simulink model "project_Auto_final"  (R2023b)
settings: Solver=FixedStepAuto  StartTime=0.0  StopTime=inf  FixedStep=0.01  RelTol=1e-3
values from neighbouring files (symbols this model uses):
  den_Gd = Gd.Den{:}    [para.m]
  encoder_scale = 1/12/4 *2*pi    (= 0.1308996939)    [para.m]
  KD = 0    [para.m]
  KI = 0.25    [para.m]
  KP = 0.05    [para.m]
  num_Gd = Gd.Num{:}    [para.m]
  Ts = 1e-2    (= 0.01)    [para.m]
  Vlim = 12    [para.m]
  Wref = 300    [para.m]
libraries: arduinolib x10, arduinosensorlib x5, simulink x2
settings Model: SimulationMode=external  ExtModeTrigDuration=2  Creator=wj671  LastModifiedBy=wj671
settings OptimizationCC: EnhancedBackFolding=on  PassReuseOutputArgsAs=Individual arguments  ZeroExternalMemoryAtStartup=off  ZeroInternalMemoryAtStartup=off  MaxStackSize=64  OptimizeBlockOrder=speed  DifferentSizesBufferReuse=on  OptimizationCustomize=off  EfficientTunableParamExpr=on
settings DebuggingCC: ParameterTunabilityLossMsg=error
settings HardwareCC: ProdBitPerInt=16  ProdBitPerPointer=16  ProdBitPerSizeT=16  ProdBitPerPtrDiffT=16  ProdLargestAtomicFloat=None  ProdWordSize=8  ProdHWDeviceType=Atmel->AVR
settings SFSimCC: MATLABDynamicMemAlloc=off
settings RTWCC: Description=Embedded Coder  SystemTargetFile=ert.tlc  HardwareBoard=Arduino Mega 2560  TemplateMakefile=ert_default_tmf  Toolchain=Arduino AVR  BuildConfiguration=Faster Runs
settings CodeAppCC: ForceParamTrailComments=on  IgnoreCustomStorageClasses=off  OperatorAnnotations=on  SimulinkDataObjDesc=on  SFDataObjDesc=on  InsertBlockDesc=on
settings ERTTargetCC: SupportContinuousTime=on  SupportVariableSizeSignals=on  ExtMode=on  ExtModeTransport=3  ExtModeStaticAlloc=on  ExtModeAutomaticAllocSize=off  ExtModeStaticAllocSize=2048  ExtModeMexFile=ext_xcp  ExtModeMexArgs=0 8 921600  ExtModeIntrfLevel=Level2 - Open

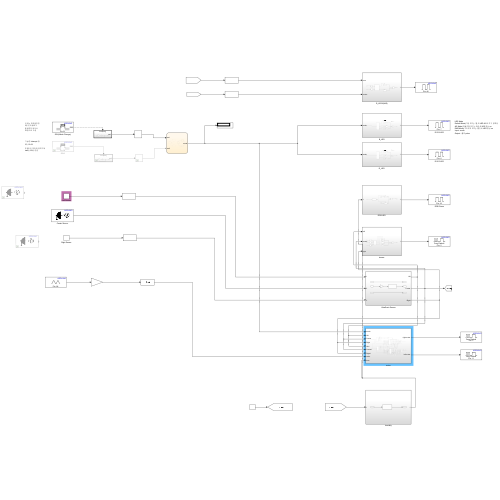
[thumbnail: Simulink's stored preview of the top-level diagram]
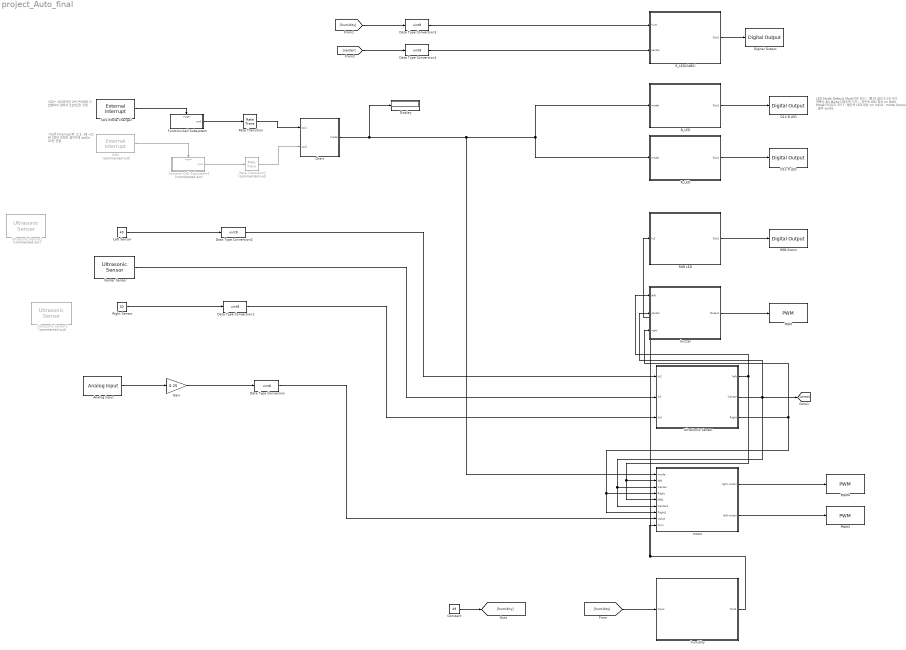
== system project_Auto_final ==
  note: 이유는 모르겠지만 2번 인터럽트가
      | 발생하지 않아서
      | 21번으로 수정
  note: 가능한 Interrupt 핀:
      | 2,3, 18~21
      |
      | 핀 3번이 모터와 겹치기에
      | sw2는 20번 연결
  note: LED Mode
      | Default Mode(기본 모드) : 빨,파 LED 0.2초 주기 깜빡임
      | AD Mode(자율주행 모드) : 파란색 LED 항상 on
      | DMS Mode(거리유지 모드) : 빨간색 LED 항상 on
      | Input : mode
      | Output : 출력 pulse
  Analog Input : arduinolib/Analog Input  pinNumber=2  ReadResultsOnly=off  ConversionTriggerSource=Software  ExternalTriggerType=uint32( 0 )  OutputDataType=uint16  EnableConversionCompleteNotify=off  EnableOuputStatus=off  SampleTime=-1  blockPlatform=arduino
  B_LED : Subsystem
  Center Sensor : arduinosensorlib/Ultrasonic Sensor  NumSignalPins=2  TrigPin=32  EchoPin=33  SignalPin=3  SampleTime_=0.1  blockPlatform=ARDUINO
  Chart : Stateflow chart  TreatAsAtomicUnit=on
  Constant : Constant  Value=49
  D12 R LED : arduinolib/Digital Output  pinNumber=6  Direction=output  blockPlatform=arduino
  D13 B LED : arduinolib/Digital Output  pinNumber=7  Direction=output  blockPlatform=arduino
  Data Type Conversion{,1..4} (5 alike) : DataTypeConversion  OutDataTypeStr=uint8  SaturateOnIntegerOverflow=off  RndMeth=Floor
  Digital Output : arduinolib/Digital Output  pinNumber=46  Direction=output  blockPlatform=arduino
  Display : Display
  Function-Call Subsystem : Subsystem  TreatAsAtomicUnit=on
  Function-Call Subsystem1 : Subsystem  Commented=on  TreatAsAtomicUnit=on
  Gain : Gain  Gain=0.25
  Left Sensor : Constant  Value=40
  PWM : arduinolib/PWM  pinNumber=5  frequencyType=Default  desiredFrequency=490.2  achievableFrequency=490.2
  PWM3 : arduinolib/PWM  pinNumber=11  frequencyType=Default  desiredFrequency=490.2  achievableFrequency=490.2
  PWM4 : arduinolib/PWM  pinNumber=3  frequencyType=Default  desiredFrequency=490.2  achievableFrequency=490.2
  RGB Grenn : arduinolib/Digital Output  pinNumber=10  Direction=output  blockPlatform=arduino
  RGB LED : Subsystem
  R_LED : Subsystem
  R_LED2(ABS) : Subsystem
  Rate Transition : RateTransition  Integrity=off  OutPortSampleTime=0.05
  Rate Transition1 : RateTransition  Commented=on  Integrity=off  OutPortSampleTime=0.05
  Right Sensor : Constant  Value=40
  SW1(Mode Change) : arduinolib/External Interrupt  Pin=21  PullUp=off  Mode=FALLING  InterruptSimulationInput=off
  SW2 : arduinolib/External Interrupt  Commented=on  Pin=20  PullUp=off  Mode=FALLING  InterruptSimulationInput=off
  UltraSonic Sensor : Subsystem
  Ultrasonic Sensor1 : arduinosensorlib/Ultrasonic Sensor  Commented=on  NumSignalPins=2  TrigPin=42  EchoPin=43  SignalPin=3  SampleTime_=0.1  blockPlatform=ARDUINO
  Ultrasonic Sensor2 : arduinosensorlib/Ultrasonic Sensor  Commented=on  NumSignalPins=2  TrigPin=50  EchoPin=51  SignalPin=3  SampleTime_=0.1  blockPlatform=ARDUINO
  buzzer : Subsystem
  humidity : Subsystem
  motor : Subsystem
  wires:
  R_LED/1(Out1) -> D12 R LED/1
  Rate Transition/1 -> Chart/1(sw1)
  B_LED/1(Out1) -> D13 B LED/1
  SW1(Mode Change)/1 -> Function-Call Subsystem/Trigger
  Function-Call Subsystem/1(sw1) -> Rate Transition/1
  Chart/1(mode) -> Display/1, motor/1(mode), B_LED/1(mode), R_LED/1(mode)
  Center Sensor/1 -> UltraSonic Sensor/2(In1)
  Left Sensor/1 -> Data Type Conversion2/1
  Right Sensor/1 -> Data Type Conversion1/1
  UltraSonic Sensor/3(Right) -> buzzer/3(right), motor/7(Right1), motor/4(Right)
  UltraSonic Sensor/1(left) -> buzzer/1(left), motor/5(left1), motor/2(left)
  UltraSonic Sensor/2(Center) -> [center], buzzer/2(center), motor/6(Center1), motor/3(Center)
  motor/1(right motor) -> PWM4/1
  motor/2(left motor) -> PWM3/1
  Data Type Conversion1/1 -> UltraSonic Sensor/3(In3)
  Data Type Conversion2/1 -> UltraSonic Sensor/1(In2)
  Function-Call Subsystem1/1(sw2) -> Rate Transition1/1
  Rate Transition1/1 -> Chart/2(sw2)
  SW2/1 -> Function-Call Subsystem1/Trigger
  Gain/1 -> Data Type Conversion/1
  Analog Input/1 -> Gain/1
  Data Type Conversion/1 -> motor/8(value)
  humidity/1(Out1) -> RGB LED/1(In2), motor/9(hum)
  RGB LED/1(Out1) -> RGB Grenn/1
  buzzer/1(Output) -> PWM/1
  Constant/1 -> [humidity]
  [humidity] -> humidity/1(Input)
  [humidity] -> Data Type Conversion3/1
  [center] -> Data Type Conversion4/1
  R_LED2(ABS)/1(Out1) -> Digital Output/1
  Data Type Conversion3/1 -> R_LED2(ABS)/1(hum)
  Data Type Conversion4/1 -> R_LED2(ABS)/2(center)

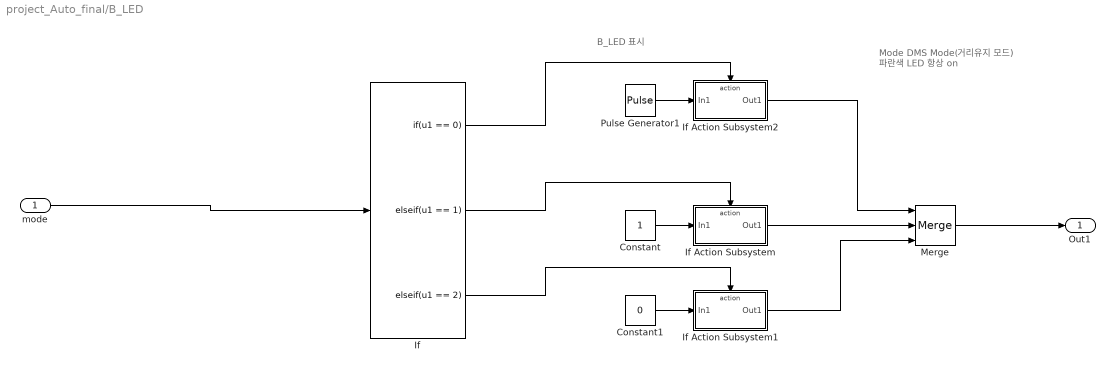
== system project_Auto_final/B_LED ==
  note: B_LED 표시
  note: Mode
      | DMS Mode(거리유지 모드)
      | 파란색 LED 항상 on
  mode : Inport
  Constant : Constant
  Constant1 : Constant  Value=0
  If : If  IfExpression=u1 == 0  ElseIfExpressions=u1 == 1, u1 == 2  ShowElse=off
  If Action Subsystem : Subsystem  TreatAsAtomicUnit=on
  If Action Subsystem1 : Subsystem  TreatAsAtomicUnit=on
  If Action Subsystem2 : Subsystem  TreatAsAtomicUnit=on
  Merge : Merge  Inputs=3
  Pulse Generator1 : DiscretePulseGenerator  PulseType=Time based  Period=0.4  PulseWidth=50
  Out1 : Outport
  wires:
  mode/1 -> If/1
  Constant/1 -> If Action Subsystem/1(In1)
  If Action Subsystem/1(Out1) -> Merge/2
  Merge/1 -> Out1/1
  If/2 -> If Action Subsystem/Action
  If/1 -> If Action Subsystem2/Action
  Pulse Generator1/1 -> If Action Subsystem2/1(In1)
  If Action Subsystem2/1(Out1) -> Merge/1
  Constant1/1 -> If Action Subsystem1/1(In1)
  If/3 -> If Action Subsystem1/Action
  If Action Subsystem1/1(Out1) -> Merge/3

== system project_Auto_final/Function-Call Subsystem ==
  function : TriggerPort  TriggerType=function-call  VariantControl=(inherit)
  Delay : Delay  DelayLength=1  InitialCondition=0
  NOT : Logic  Operator=NOT  IconShape=distinctive  AllPortsSameDT=off  OutDataTypeStr=boolean
  sw1 : Outport
  wires:
  Delay/1 -> NOT/1
  NOT/1 -> Delay/1, sw1/1

== system project_Auto_final/Function-Call Subsystem1 ==
  function : TriggerPort  TriggerType=function-call  VariantControl=(inherit)
  Delay : Delay  DelayLength=1  InitialCondition=0
  NOT : Logic  Operator=NOT  IconShape=distinctive  AllPortsSameDT=off  OutDataTypeStr=boolean
  sw2 : Outport
  wires:
  Delay/1 -> NOT/1
  NOT/1 -> Delay/1, sw2/1

== system project_Auto_final/RGB LED ==
  In2 : Inport
  Constant : Constant  Value=0
  If : If  IfExpression=u1 > 50
  If Action Subsystem : Subsystem  TreatAsAtomicUnit=on
  If Action Subsystem1 : Subsystem  TreatAsAtomicUnit=on
  Merge : Merge
  Pulse Generator : DiscretePulseGenerator  PulseType=Time based  Period=4  PulseWidth=50
  Out1 : Outport
  wires:
  In2/1 -> If/1
  If/1 -> If Action Subsystem/Action
  If/2 -> If Action Subsystem1/Action
  Pulse Generator/1 -> If Action Subsystem/1(In1)
  Constant/1 -> If Action Subsystem1/1(In1)
  If Action Subsystem/1(Out1) -> Merge/1
  If Action Subsystem1/1(Out1) -> Merge/2
  Merge/1 -> Out1/1

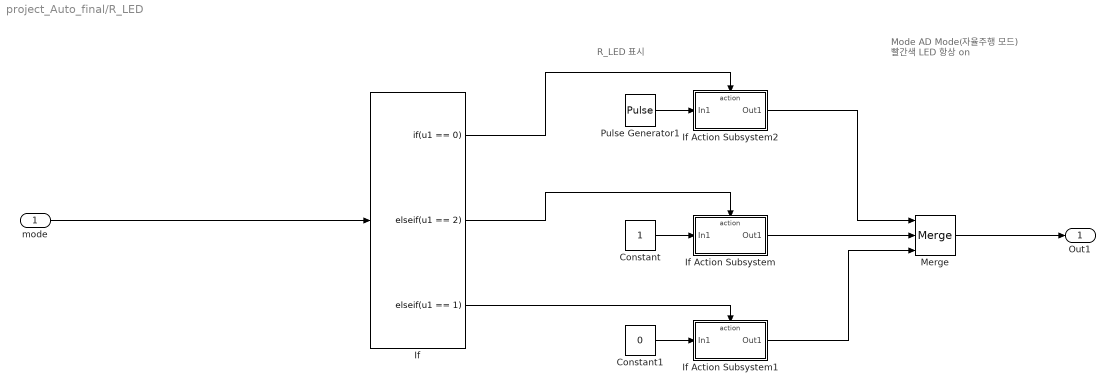
== system project_Auto_final/R_LED ==
  note: R_LED 표시
  note: Mode
      | AD Mode(자율주행 모드)
      | 빨간색 LED 항상 on
  mode : Inport
  Constant : Constant
  Constant1 : Constant  Value=0
  If : If  IfExpression=u1 == 0  ElseIfExpressions=u1 == 2, u1 == 1  ShowElse=off
  If Action Subsystem : Subsystem  TreatAsAtomicUnit=on
  If Action Subsystem1 : Subsystem  TreatAsAtomicUnit=on
  If Action Subsystem2 : Subsystem  TreatAsAtomicUnit=on
  Merge : Merge  Inputs=3
  Pulse Generator1 : DiscretePulseGenerator  PulseType=Time based  Period=0.4  PulseWidth=50
  Out1 : Outport
  wires:
  mode/1 -> If/1
  Constant/1 -> If Action Subsystem/1(In1)
  If Action Subsystem/1(Out1) -> Merge/2
  Merge/1 -> Out1/1
  If/2 -> If Action Subsystem/Action
  If/1 -> If Action Subsystem2/Action
  Pulse Generator1/1 -> If Action Subsystem2/1(In1)
  If Action Subsystem2/1(Out1) -> Merge/1
  If/3 -> If Action Subsystem1/Action
  Constant1/1 -> If Action Subsystem1/1(In1)
  If Action Subsystem1/1(Out1) -> Merge/3

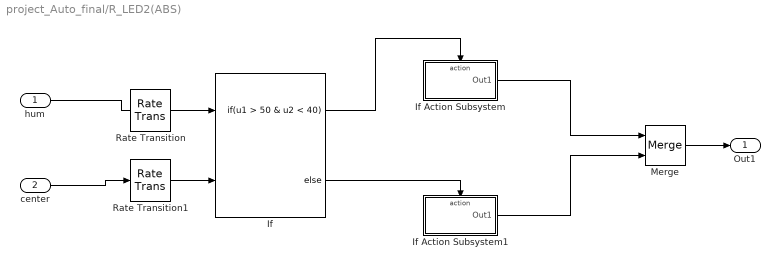
== system project_Auto_final/R_LED2(ABS) ==
  hum : Inport
  center : Inport  Port=2
  If : If  NumInputs=2  IfExpression=u1 > 50 & u2 < 40
  If Action Subsystem : Subsystem  TreatAsAtomicUnit=on
  If Action Subsystem1 : Subsystem  TreatAsAtomicUnit=on
  Merge : Merge
  Rate Transition : RateTransition  Integrity=off
  Rate Transition1 : RateTransition  Integrity=off
  Out1 : Outport
  wires:
  hum/1 -> If/1
  center/1 -> Rate Transition1/1
  Merge/1 -> Out1/1
  If/1 -> If Action Subsystem/Action
  If Action Subsystem/1(Out1) -> Merge/1
  If/2 -> If Action Subsystem1/Action
  If Action Subsystem1/1(Out1) -> Merge/2
  Rate Transition1/1 -> If/2

== system project_Auto_final/UltraSonic Sensor ==
  In2 : Inport
  In1 : Inport  Port=2
  In3 : Inport  Port=3
  Data Type Conversion : DataTypeConversion  OutDataTypeStr=uint8  SaturateOnIntegerOverflow=off  RndMeth=Floor
  Gain : Gain  Gain=100
  left : Outport
  Center : Outport  Port=2
  Right : Outport  Port=3
  wires:
  In1/1 -> Gain/1
  Gain/1 -> Data Type Conversion/1
  Data Type Conversion/1 -> Center/1
  In3/1 -> Right/1
  In2/1 -> left/1

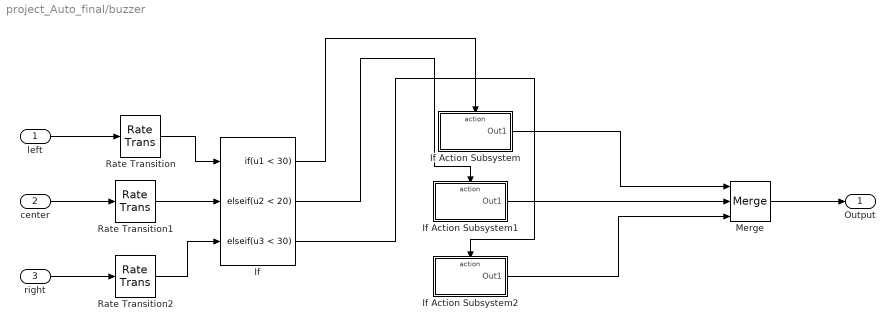
== system project_Auto_final/buzzer ==
  left : Inport
  center : Inport  Port=2
  right : Inport  Port=3
  If : If  NumInputs=3  IfExpression=u1 < 30  ElseIfExpressions=u2 < 20, u3 < 30  ShowElse=off
  If Action Subsystem : Subsystem  TreatAsAtomicUnit=on
  If Action Subsystem1 : Subsystem  TreatAsAtomicUnit=on
  If Action Subsystem2 : Subsystem  TreatAsAtomicUnit=on
  Merge : Merge  Inputs=3
  Rate Transition : RateTransition  Integrity=off
  Rate Transition1 : RateTransition  Integrity=off
  Rate Transition2 : RateTransition  Integrity=off
  Output : Outport
  wires:
  Merge/1 -> Output/1
  left/1 -> Rate Transition/1
  center/1 -> Rate Transition1/1
  right/1 -> Rate Transition2/1
  If/1 -> If Action Subsystem/Action
  If/2 -> If Action Subsystem1/Action
  If/3 -> If Action Subsystem2/Action
  If Action Subsystem/1(Out1) -> Merge/1
  If Action Subsystem1/1(Out1) -> Merge/2
  If Action Subsystem2/1(Out1) -> Merge/3
  Rate Transition/1 -> If/1
  Rate Transition1/1 -> If/2
  Rate Transition2/1 -> If/3

== system project_Auto_final/humidity ==
  Input : Inport
  Data Type Conversion : DataTypeConversion  OutDataTypeStr=uint8  SaturateOnIntegerOverflow=off  RndMeth=Floor
  Out1 : Outport
  wires:
  Input/1 -> Data Type Conversion/1
  Data Type Conversion/1 -> Out1/1

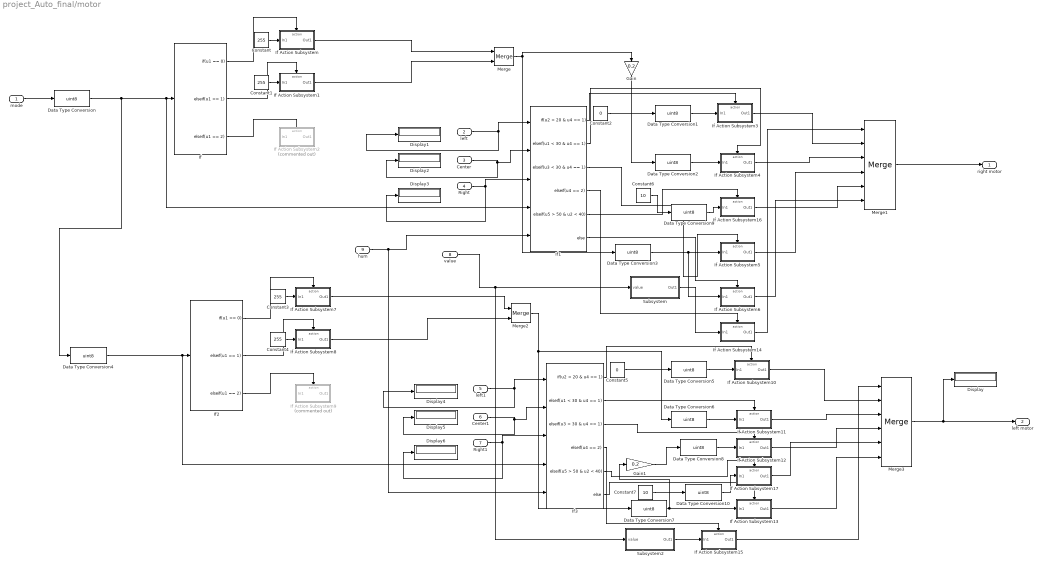
== system project_Auto_final/motor ==
  mode : Inport
  left : Inport  Port=2
  Center : Inport  Port=3
  Right : Inport  Port=4
  left1 : Inport  Port=5
  Center1 : Inport  Port=6
  Right1 : Inport  Port=7
  value : Inport  Port=8
  hum : Inport  Port=9
  Constant{,1,3..4} (4 alike) : Constant  Value=255
  Constant2 : Constant  Value=0
  Constant5 : Constant  Value=0
  Constant6 : Constant  Value=10
  Constant7 : Constant  Value=10
  Data Type Conversion{,1..10} (11 alike) : DataTypeConversion  OutDataTypeStr=uint8  SaturateOnIntegerOverflow=off  RndMeth=Floor
  Display{,1..6} (7 alike) : Display
  Gain : Gain  Gain=0.2
  Gain1 : Gain  Gain=0.2
  If : If  IfExpression=u1 == 0  ElseIfExpressions=u1 == 1, u1 == 2  ShowElse=off
  If Action Subsystem : Subsystem  TreatAsAtomicUnit=on
  If Action Subsystem1 : Subsystem  TreatAsAtomicUnit=on
  If Action Subsystem10 : Subsystem  TreatAsAtomicUnit=on
  If Action Subsystem11 : Subsystem  TreatAsAtomicUnit=on
  If Action Subsystem12 : Subsystem  TreatAsAtomicUnit=on
  If Action Subsystem13 : Subsystem  TreatAsAtomicUnit=on
  If Action Subsystem14 : Subsystem  TreatAsAtomicUnit=on
  If Action Subsystem15 : Subsystem  TreatAsAtomicUnit=on
  If Action Subsystem16 : Subsystem  TreatAsAtomicUnit=on
  If Action Subsystem17 : Subsystem  TreatAsAtomicUnit=on
  If Action Subsystem2 : Subsystem  Commented=on  TreatAsAtomicUnit=on
  If Action Subsystem3 : Subsystem  TreatAsAtomicUnit=on
  If Action Subsystem4 : Subsystem  TreatAsAtomicUnit=on
  If Action Subsystem5 : Subsystem  TreatAsAtomicUnit=on
  If Action Subsystem6 : Subsystem  TreatAsAtomicUnit=on
  If Action Subsystem7 : Subsystem  TreatAsAtomicUnit=on
  If Action Subsystem8 : Subsystem  TreatAsAtomicUnit=on
  If Action Subsystem9 : Subsystem  Commented=on  TreatAsAtomicUnit=on
  If1 : If  NumInputs=5  IfExpression=u2 < 20 & u4 == 1  ElseIfExpressions=u1 < 30 & u4 == 1, u3 < 30 & u4 == 1, u4 == 2, u5 > 50 & u2 < 40
  If2 : If  IfExpression=u1 == 0  ElseIfExpressions=u1 == 1, u1 == 2  ShowElse=off
  If3 : If  NumInputs=5  IfExpression=u2 < 20 & u4 == 1  ElseIfExpressions=u1 < 30 & u4 == 1, u3 < 30 & u4 == 1, u4 == 2, u5 > 50 & u2 < 40
  Merge : Merge
  Merge1 : Merge  Inputs=6
  Merge2 : Merge
  Merge3 : Merge  Inputs=6
  Subsystem : Subsystem
  Subsystem2 : Subsystem
  right motor : Outport
  left motor : Outport  Port=2
  wires:
  mode/1 -> Data Type Conversion/1
  If/1 -> If Action Subsystem/Action
  If/2 -> If Action Subsystem1/Action
  If/3 -> If Action Subsystem2/Action
  Constant/1 -> If Action Subsystem/1(In1)
  Constant1/1 -> If Action Subsystem1/1(In1)
  If Action Subsystem/1(Out1) -> Merge/1
  If Action Subsystem1/1(Out1) -> Merge/2
  left/1 -> Display1/1, If1/1
  Center/1 -> Display2/1, If1/2
  Right/1 -> Display3/1, If1/3
  If1/3 -> If Action Subsystem5/Action
  If1/6 -> If Action Subsystem6/Action
  Merge/1 -> Data Type Conversion3/1, Gain/1
  If1/1 -> If Action Subsystem3/Action
  If1/2 -> If Action Subsystem4/Action
  Constant2/1 -> Data Type Conversion1/1
  Gain/1 -> Data Type Conversion2/1
  If Action Subsystem3/1(Out1) -> Merge1/2
  If Action Subsystem4/1(Out1) -> Merge1/3
  If Action Subsystem5/1(Out1) -> Merge1/4
  If Action Subsystem6/1(Out1) -> Merge1/6
  Merge1/1 -> right motor/1
  Data Type Conversion1/1 -> If Action Subsystem3/1(In1)
  Data Type Conversion2/1 -> If Action Subsystem4/1(In1)
  Data Type Conversion3/1 -> If Action Subsystem5/1(In1), If Action Subsystem6/1(In1)
  Constant3/1 -> If Action Subsystem7/1(In1)
  If Action Subsystem8/1(Out1) -> Merge2/2
  Data Type Conversion6/1 -> If Action Subsystem11/1(In1)
  If2/2 -> If Action Subsystem8/Action
  If2/1 -> If Action Subsystem7/Action
  If3/1 -> If Action Subsystem10/Action
  If Action Subsystem7/1(Out1) -> Merge2/1
  Merge3/1 -> Display/1, left motor/1
  left1/1 -> Display4/1, If3/1
  If Action Subsystem10/1(Out1) -> Merge3/2
  Constant5/1 -> Data Type Conversion5/1
  If2/3 -> If Action Subsystem9/Action
  If3/2 -> If Action Subsystem11/Action
  Data Type Conversion/1 -> Data Type Conversion4/1, If1/4, If/1
  Data Type Conversion7/1 -> If Action Subsystem13/1(In1), Gain1/1
  Data Type Conversion4/1 -> If3/4, If2/1
  Center1/1 -> Display5/1, If3/2
  If Action Subsystem12/1(Out1) -> Merge3/4
  Constant4/1 -> If Action Subsystem8/1(In1)
  If3/6 -> If Action Subsystem13/Action
  Data Type Conversion5/1 -> If Action Subsystem10/1(In1)
  If Action Subsystem11/1(Out1) -> Merge3/3
  Right1/1 -> Display6/1, If3/3
  Merge2/1 -> Data Type Conversion6/1, Data Type Conversion7/1
  If Action Subsystem13/1(Out1) -> Merge3/6
  If3/3 -> If Action Subsystem12/Action
  Gain1/1 -> Data Type Conversion8/1
  Data Type Conversion8/1 -> If Action Subsystem12/1(In1)
  If1/4 -> If Action Subsystem14/Action
  Subsystem/1(Out1) -> If Action Subsystem14/1(In1)
  If Action Subsystem14/1(Out1) -> Merge1/1
  If3/4 -> If Action Subsystem15/Action
  If Action Subsystem15/1(Out1) -> Merge3/1
  value/1 -> Subsystem2/1(value), Subsystem/1(value)
  Subsystem2/1(Out1) -> If Action Subsystem15/1(In1)
  hum/1 -> If3/5, If1/5
  If1/5 -> If Action Subsystem16/Action
  Constant6/1 -> Data Type Conversion9/1
  Data Type Conversion9/1 -> If Action Subsystem16/1(In1)
  If Action Subsystem16/1(Out1) -> Merge1/5
  If3/5 -> If Action Subsystem17/Action
  Constant7/1 -> Data Type Conversion10/1
  Data Type Conversion10/1 -> If Action Subsystem17/1(In1)
  If Action Subsystem17/1(Out1) -> Merge3/5

== system project_Auto_final/B_LED/If Action Subsystem ==
  In1 : Inport
  Action Port : ActionPort  ActionPortLabel=elseif(u1 == 1)
  Out1 : Outport
  wires:
  In1/1 -> Out1/1

== system project_Auto_final/B_LED/If Action Subsystem1 ==
  In1 : Inport
  Action Port : ActionPort  ActionPortLabel=elseif( u1 == 2)
  Out1 : Outport
  wires:
  In1/1 -> Out1/1

== system project_Auto_final/B_LED/If Action Subsystem2 ==
  In1 : Inport
  Action Port : ActionPort  ActionPortLabel=if(u1 == 0)
  Out1 : Outport
  wires:
  In1/1 -> Out1/1

== system project_Auto_final/RGB LED/If Action Subsystem ==
  In1 : Inport
  Action Port : ActionPort  ActionPortLabel=if(u1 > 50)
  Out1 : Outport
  wires:
  In1/1 -> Out1/1

== system project_Auto_final/RGB LED/If Action Subsystem1 ==
  In1 : Inport
  Action Port : ActionPort  ActionPortLabel=else
  Out1 : Outport
  wires:
  In1/1 -> Out1/1

== system project_Auto_final/R_LED/If Action Subsystem ==
  In1 : Inport
  Action Port : ActionPort  ActionPortLabel=elseif(u1 == 2)
  Out1 : Outport
  wires:
  In1/1 -> Out1/1

== system project_Auto_final/R_LED/If Action Subsystem1 ==
  In1 : Inport
  Action Port : ActionPort  ActionPortLabel=elseif( u1 == 1)
  Out1 : Outport
  wires:
  In1/1 -> Out1/1

== system project_Auto_final/R_LED/If Action Subsystem2 ==
  In1 : Inport
  Action Port : ActionPort  ActionPortLabel=if(u1 == 0)
  Out1 : Outport
  wires:
  In1/1 -> Out1/1

== system project_Auto_final/R_LED2(ABS)/If Action Subsystem ==
  Action Port : ActionPort  ActionPortLabel=if(u1 > 50 & u2 < 40)
  Pulse Generator : DiscretePulseGenerator  PulseType=Time based  Period=0.2  PulseWidth=50
  Out1 : Outport
  wires:
  Pulse Generator/1 -> Out1/1

== system project_Auto_final/R_LED2(ABS)/If Action Subsystem1 ==
  Action Port : ActionPort  ActionPortLabel=else
  Constant : Constant  Value=0
  Out1 : Outport
  wires:
  Constant/1 -> Out1/1

== system project_Auto_final/buzzer/If Action Subsystem ==
  Action Port : ActionPort  ActionPortLabel=if(u1 < 30)
  Pulse Generator : DiscretePulseGenerator  PulseType=Time based  Amplitude=200  Period=4  PulseWidth=50
  Out1 : Outport
  wires:
  Pulse Generator/1 -> Out1/1

== system project_Auto_final/buzzer/If Action Subsystem1 ==
  Action Port : ActionPort  ActionPortLabel=elseif(u2 < 20)
  Pulse Generator : DiscretePulseGenerator  PulseType=Time based  Amplitude=200  Period=6  PulseWidth=50
  Out1 : Outport
  wires:
  Pulse Generator/1 -> Out1/1

== system project_Auto_final/buzzer/If Action Subsystem2 ==
  Action Port : ActionPort  ActionPortLabel=elseif( u3 < 30)
  Pulse Generator : DiscretePulseGenerator  PulseType=Time based  Amplitude=200  Period=4  PulseWidth=50
  Out1 : Outport
  wires:
  Pulse Generator/1 -> Out1/1

== system project_Auto_final/motor/If Action Subsystem ==
  In1 : Inport
  Action Port : ActionPort  ActionPortLabel=if(u1 == 0)
  Out1 : Outport
  wires:
  In1/1 -> Out1/1

== system project_Auto_final/motor/If Action Subsystem1 ==
  In1 : Inport
  Action Port : ActionPort  ActionPortLabel=elseif(u1 == 1)
  Out1 : Outport
  wires:
  In1/1 -> Out1/1

== system project_Auto_final/motor/If Action Subsystem10 ==
  In1 : Inport
  Action Port : ActionPort  ActionPortLabel=if(u2 < 20 & u4 == 1)
  Out1 : Outport
  wires:
  In1/1 -> Out1/1

== system project_Auto_final/motor/If Action Subsystem11 ==
  In1 : Inport
  Action Port : ActionPort  ActionPortLabel=elseif(u1 < 30 & u4 == 1)
  Out1 : Outport
  wires:
  In1/1 -> Out1/1

== system project_Auto_final/motor/If Action Subsystem12 ==
  In1 : Inport
  Action Port : ActionPort  ActionPortLabel=elseif( u3 < 30 & u4 == 1)
  Out1 : Outport
  wires:
  In1/1 -> Out1/1

== system project_Auto_final/motor/If Action Subsystem13 ==
  In1 : Inport
  Action Port : ActionPort  ActionPortLabel=else
  Out1 : Outport
  wires:
  In1/1 -> Out1/1

== system project_Auto_final/motor/If Action Subsystem14 ==
  In1 : Inport
  Action Port : ActionPort  ActionPortLabel=elseif( u4 == 2)
  Out1 : Outport
  wires:
  In1/1 -> Out1/1

== system project_Auto_final/motor/If Action Subsystem15 ==
  In1 : Inport
  Action Port : ActionPort  ActionPortLabel=elseif( u4 == 2)
  Out1 : Outport
  wires:
  In1/1 -> Out1/1

== system project_Auto_final/motor/If Action Subsystem16 ==
  In1 : Inport
  Action Port : ActionPort  ActionPortLabel=elseif( u5 > 50 & u2 < 40)
  Out1 : Outport
  wires:
  In1/1 -> Out1/1

== system project_Auto_final/motor/If Action Subsystem17 ==
  In1 : Inport
  Action Port : ActionPort  ActionPortLabel=elseif( u5 > 50 & u2 < 40)
  Out1 : Outport
  wires:
  In1/1 -> Out1/1

== system project_Auto_final/motor/If Action Subsystem2 ==
  In1 : Inport
  Action Port : ActionPort  ActionPortLabel=elseif( u1 == 2)
  Out1 : Outport
  wires:
  In1/1 -> Out1/1

== system project_Auto_final/motor/If Action Subsystem3 ==
  In1 : Inport
  Action Port : ActionPort  ActionPortLabel=if(u2 < 20 & u4 == 1)
  Out1 : Outport
  wires:
  In1/1 -> Out1/1

== system project_Auto_final/motor/If Action Subsystem4 ==
  In1 : Inport
  Action Port : ActionPort  ActionPortLabel=elseif(u1 < 30 & u4 == 1)
  Out1 : Outport
  wires:
  In1/1 -> Out1/1

== system project_Auto_final/motor/If Action Subsystem5 ==
  In1 : Inport
  Action Port : ActionPort  ActionPortLabel=elseif( u3 < 30 & u4 == 1)
  Out1 : Outport
  wires:
  In1/1 -> Out1/1

== system project_Auto_final/motor/If Action Subsystem6 ==
  In1 : Inport
  Action Port : ActionPort  ActionPortLabel=else
  Out1 : Outport
  wires:
  In1/1 -> Out1/1

== system project_Auto_final/motor/If Action Subsystem7 ==
  In1 : Inport
  Action Port : ActionPort  ActionPortLabel=if(u1 == 0)
  Out1 : Outport
  wires:
  In1/1 -> Out1/1

== system project_Auto_final/motor/If Action Subsystem8 ==
  In1 : Inport
  Action Port : ActionPort  ActionPortLabel=elseif(u1 == 1)
  Out1 : Outport
  wires:
  In1/1 -> Out1/1

== system project_Auto_final/motor/If Action Subsystem9 ==
  In1 : Inport
  Action Port : ActionPort  ActionPortLabel=elseif( u1 == 2)
  Out1 : Outport
  wires:
  In1/1 -> Out1/1

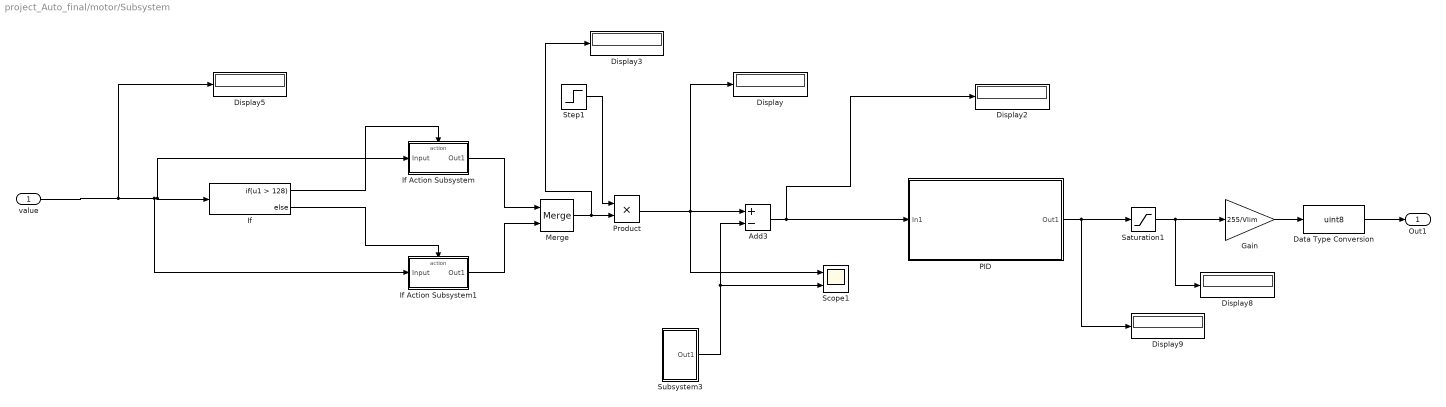
== system project_Auto_final/motor/Subsystem ==
  value : Inport
  Add3 : Sum  Inputs=+-
  Data Type Conversion : DataTypeConversion  OutDataTypeStr=uint8  SaturateOnIntegerOverflow=off  RndMeth=Floor
  Display{,2..3,5,8..9} (6 alike) : Display
  Gain : Gain  Gain=255/Vlim
  If : If  IfExpression=u1 > 128
  If Action Subsystem : Subsystem  TreatAsAtomicUnit=on
  If Action Subsystem1 : Subsystem  TreatAsAtomicUnit=on
  Merge : Merge
  PID : Subsystem
  Product : Product
  Saturation1 : Saturate  UpperLimit=12  LowerLimit=0
  Scope1 : Scope  NumInputPorts=2
  Step1 : Step  After=Wref  SampleTime=0
  Subsystem3 : Subsystem
  Out1 : Outport
  wires:
  If Action Subsystem1/1(Out1) -> Merge/2
  If/1 -> If Action Subsystem/Action
  Gain/1 -> Data Type Conversion/1
  Subsystem3/1(Out1) -> Scope1/2, Add3/2
  If/2 -> If Action Subsystem1/Action
  Add3/1 -> Display2/1, PID/1(In1)
  Merge/1 -> Display3/1, Product/2
  Product/1 -> Scope1/1, Add3/1, Display/1
  PID/1(Out1) -> Display9/1, Saturation1/1
  Step1/1 -> Product/1
  If Action Subsystem/1(Out1) -> Merge/1
  Saturation1/1 -> Gain/1, Display8/1
  value/1 -> Display5/1, If Action Subsystem1/1(Input), If/1, If Action Subsystem/1(Input)
  Data Type Conversion/1 -> Out1/1

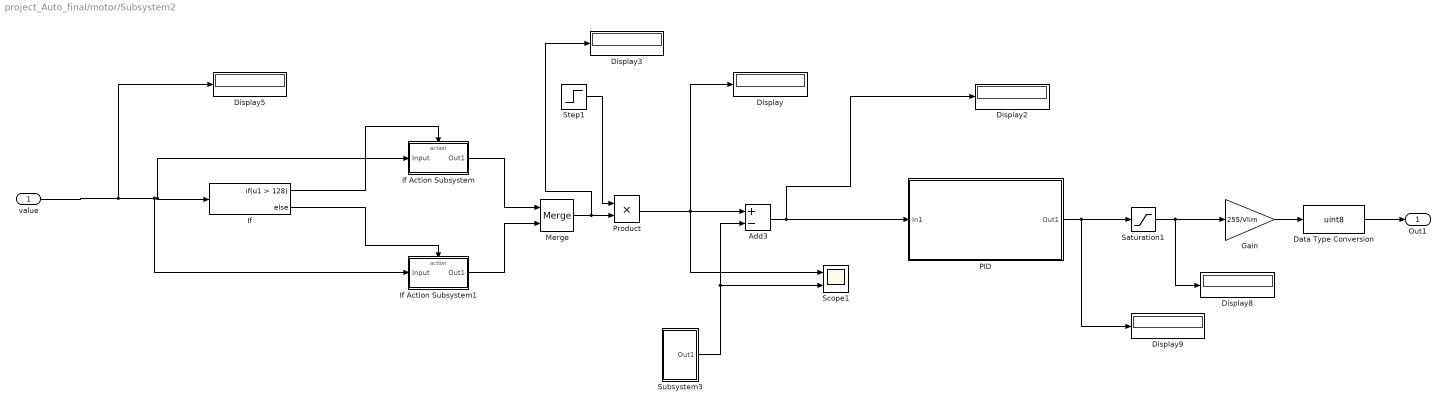
== system project_Auto_final/motor/Subsystem2 ==
  value : Inport
  Add3 : Sum  Inputs=+-
  Data Type Conversion : DataTypeConversion  OutDataTypeStr=uint8  SaturateOnIntegerOverflow=off  RndMeth=Floor
  Display{,2..3,5,8..9} (6 alike) : Display
  Gain : Gain  Gain=255/Vlim
  If : If  IfExpression=u1 > 128
  If Action Subsystem : Subsystem  TreatAsAtomicUnit=on
  If Action Subsystem1 : Subsystem  TreatAsAtomicUnit=on
  Merge : Merge
  PID : Subsystem
  Product : Product
  Saturation1 : Saturate  UpperLimit=12  LowerLimit=0
  Scope1 : Scope  NumInputPorts=2
  Step1 : Step  After=Wref  SampleTime=0
  Subsystem3 : Subsystem
  Out1 : Outport
  wires:
  If Action Subsystem1/1(Out1) -> Merge/2
  If/1 -> If Action Subsystem/Action
  Gain/1 -> Data Type Conversion/1
  Subsystem3/1(Out1) -> Scope1/2, Add3/2
  If/2 -> If Action Subsystem1/Action
  Add3/1 -> Display2/1, PID/1(In1)
  Merge/1 -> Display3/1, Product/2
  Product/1 -> Scope1/1, Add3/1, Display/1
  PID/1(Out1) -> Display9/1, Saturation1/1
  Step1/1 -> Product/1
  If Action Subsystem/1(Out1) -> Merge/1
  Saturation1/1 -> Gain/1, Display8/1
  value/1 -> Display5/1, If Action Subsystem1/1(Input), If/1, If Action Subsystem/1(Input)
  Data Type Conversion/1 -> Out1/1

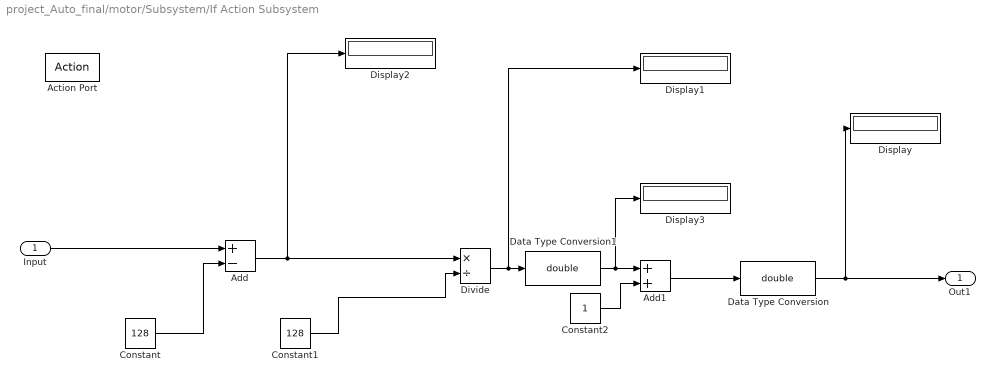
== system project_Auto_final/motor/Subsystem/If Action Subsystem ==
  Input : Inport
  Action Port : ActionPort  ActionPortLabel=if(u1 > 128)
  Add : Sum  Inputs=+-
  Add1 : Sum
  Constant : Constant  Value=128
  Constant1 : Constant  Value=128
  Constant2 : Constant
  Data Type Conversion : DataTypeConversion  OutDataTypeStr=double  SaturateOnIntegerOverflow=off  RndMeth=Floor
  Data Type Conversion1 : DataTypeConversion  OutDataTypeStr=double  SaturateOnIntegerOverflow=off  RndMeth=Floor
  Display{,1..3} (4 alike) : Display
  Divide : Product  Inputs=*/
  Out1 : Outport
  wires:
  Constant1/1 -> Divide/2
  Input/1 -> Add/1
  Constant/1 -> Add/2
  Constant2/1 -> Add1/2
  Add1/1 -> Data Type Conversion/1
  Data Type Conversion/1 -> Display/1, Out1/1
  Add/1 -> Divide/1, Display2/1
  Divide/1 -> Display1/1, Data Type Conversion1/1
  Data Type Conversion1/1 -> Display3/1, Add1/1

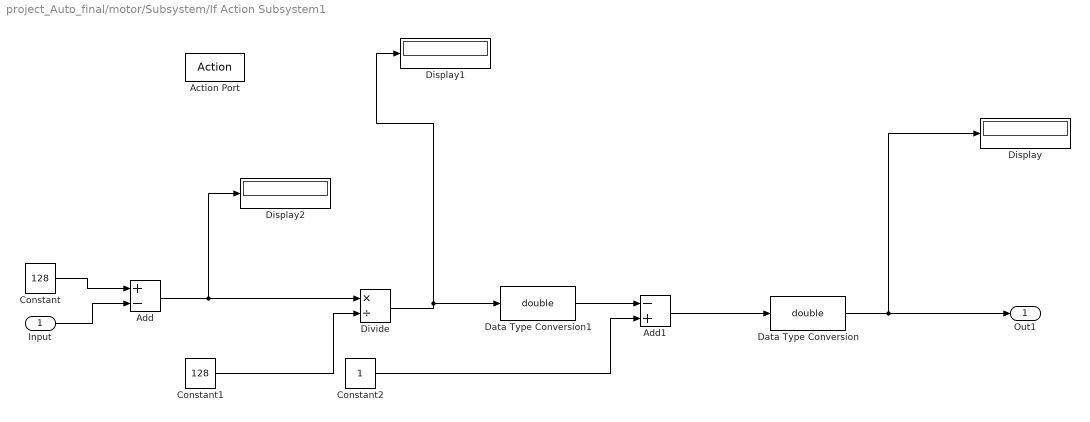
== system project_Auto_final/motor/Subsystem/If Action Subsystem1 ==
  Input : Inport
  Action Port : ActionPort  ActionPortLabel=else
  Add : Sum  Inputs=+-
  Add1 : Sum  Inputs=-+
  Constant : Constant  Value=128
  Constant1 : Constant  Value=128
  Constant2 : Constant
  Data Type Conversion : DataTypeConversion  OutDataTypeStr=double  SaturateOnIntegerOverflow=off  RndMeth=Floor
  Data Type Conversion1 : DataTypeConversion  OutDataTypeStr=double  SaturateOnIntegerOverflow=off  RndMeth=Floor
  Display : Display
  Display1 : Display
  Display2 : Display
  Divide : Product  Inputs=*/
  Out1 : Outport
  wires:
  Constant2/1 -> Add1/2
  Constant1/1 -> Divide/2
  Add1/1 -> Data Type Conversion/1
  Data Type Conversion/1 -> Display/1, Out1/1
  Constant/1 -> Add/1
  Input/1 -> Add/2
  Divide/1 -> Data Type Conversion1/1, Display1/1
  Add/1 -> Divide/1, Display2/1
  Data Type Conversion1/1 -> Add1/1

== system project_Auto_final/motor/Subsystem/PID ==
  In1 : Inport
  Derivative2 : Derivative
  Gain1 : Gain  Gain=KI
  Gain2 : Gain  Gain=KP
  Gain3 : Gain  Gain=KD
  Integrator2 : Integrator
  Subtract2 : Sum  Inputs=+++
  Out1 : Outport
  wires:
  Gain1/1 -> Integrator2/1
  Gain2/1 -> Subtract2/2
  Integrator2/1 -> Subtract2/1
  In1/1 -> Gain2/1, Gain3/1, Gain1/1
  Derivative2/1 -> Subtract2/3
  Gain3/1 -> Derivative2/1
  Subtract2/1 -> Out1/1

== system project_Auto_final/motor/Subsystem/Subsystem3 ==
  Data Type Conversion1 : DataTypeConversion  OutDataTypeStr=int32  SaturateOnIntegerOverflow=off  RndMeth=Floor
  Discrete Transfer Fcn : DiscreteTransferFcn  Numerator=num_Gd  Denominator=den_Gd  SampleTime=Ts
  Discrete Derivative : simulink/Discrete/Discrete Derivative  gainval=1.0  ICPrevScaledInput=0.0  InputProcessing=Columns as channels (frame based)  OutMin=[]  OutMax=[]  OutDataType=fixdt(1, 16)  OutScaling=2^-10  DoSatur=off
  Display : Display
  Display1 : Display
  Encoder : arduinosensorlib/Encoder  InputA=18  InputB=19  Mode=No reset  SampleTime=-1
  Gain1 : Gain  Gain=encoder_scale
  Gain2 : Gain  Gain=60/(2*pi)
  Out1 : Outport
  wires:
  Gain1/1 -> Gain2/1, Display/1, Data Type Conversion1/1
  Encoder/1 -> Discrete Derivative/1
  Gain2/1 -> Display1/1
  Discrete Derivative/1 -> Gain1/1
  Discrete Transfer Fcn/1 -> Out1/1  "W(rad/s)"
  Data Type Conversion1/1 -> Discrete Transfer Fcn/1

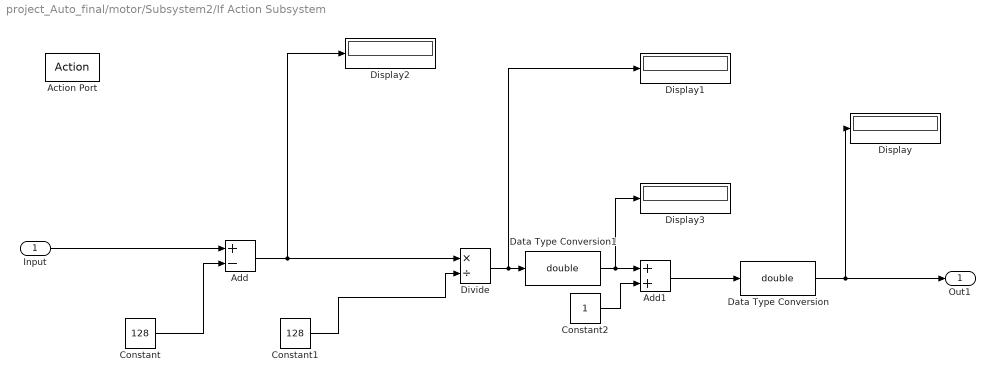
== system project_Auto_final/motor/Subsystem2/If Action Subsystem ==
  Input : Inport
  Action Port : ActionPort  ActionPortLabel=if(u1 > 128)
  Add : Sum  Inputs=+-
  Add1 : Sum
  Constant : Constant  Value=128
  Constant1 : Constant  Value=128
  Constant2 : Constant
  Data Type Conversion : DataTypeConversion  OutDataTypeStr=double  SaturateOnIntegerOverflow=off  RndMeth=Floor
  Data Type Conversion1 : DataTypeConversion  OutDataTypeStr=double  SaturateOnIntegerOverflow=off  RndMeth=Floor
  Display{,1..3} (4 alike) : Display
  Divide : Product  Inputs=*/
  Out1 : Outport
  wires:
  Constant1/1 -> Divide/2
  Input/1 -> Add/1
  Constant/1 -> Add/2
  Constant2/1 -> Add1/2
  Add1/1 -> Data Type Conversion/1
  Data Type Conversion/1 -> Display/1, Out1/1
  Add/1 -> Divide/1, Display2/1
  Divide/1 -> Display1/1, Data Type Conversion1/1
  Data Type Conversion1/1 -> Display3/1, Add1/1

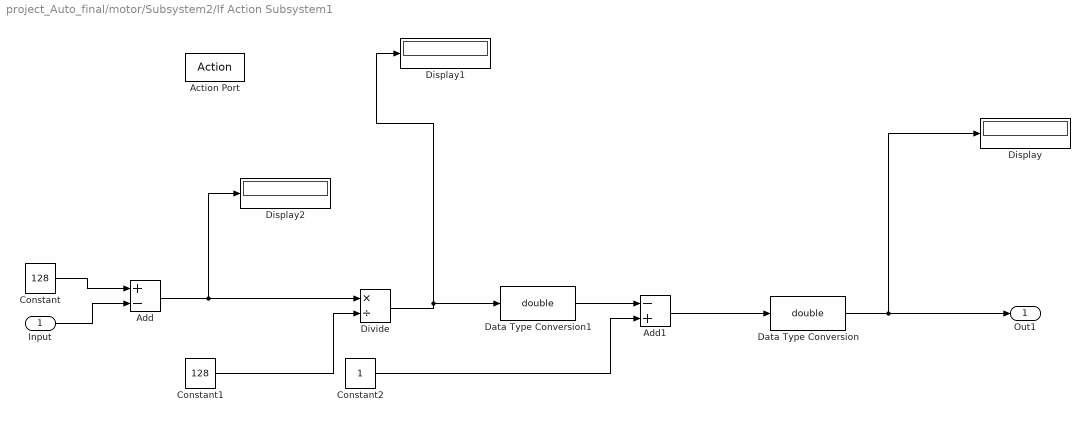
== system project_Auto_final/motor/Subsystem2/If Action Subsystem1 ==
  Input : Inport
  Action Port : ActionPort  ActionPortLabel=else
  Add : Sum  Inputs=+-
  Add1 : Sum  Inputs=-+
  Constant : Constant  Value=128
  Constant1 : Constant  Value=128
  Constant2 : Constant
  Data Type Conversion : DataTypeConversion  OutDataTypeStr=double  SaturateOnIntegerOverflow=off  RndMeth=Floor
  Data Type Conversion1 : DataTypeConversion  OutDataTypeStr=double  SaturateOnIntegerOverflow=off  RndMeth=Floor
  Display : Display
  Display1 : Display
  Display2 : Display
  Divide : Product  Inputs=*/
  Out1 : Outport
  wires:
  Constant2/1 -> Add1/2
  Constant1/1 -> Divide/2
  Add1/1 -> Data Type Conversion/1
  Data Type Conversion/1 -> Display/1, Out1/1
  Constant/1 -> Add/1
  Input/1 -> Add/2
  Divide/1 -> Data Type Conversion1/1, Display1/1
  Add/1 -> Divide/1, Display2/1
  Data Type Conversion1/1 -> Add1/1

== system project_Auto_final/motor/Subsystem2/PID ==
  In1 : Inport
  Derivative2 : Derivative
  Gain1 : Gain  Gain=KI
  Gain2 : Gain  Gain=KP
  Gain3 : Gain  Gain=KD
  Integrator2 : Integrator
  Subtract2 : Sum  Inputs=+++
  Out1 : Outport
  wires:
  Gain1/1 -> Integrator2/1
  Gain2/1 -> Subtract2/2
  Integrator2/1 -> Subtract2/1
  In1/1 -> Gain2/1, Gain3/1, Gain1/1
  Derivative2/1 -> Subtract2/3
  Gain3/1 -> Derivative2/1
  Subtract2/1 -> Out1/1

== system project_Auto_final/motor/Subsystem2/Subsystem3 ==
  Data Type Conversion1 : DataTypeConversion  OutDataTypeStr=int32  SaturateOnIntegerOverflow=off  RndMeth=Floor
  Discrete Transfer Fcn : DiscreteTransferFcn  Numerator=num_Gd  Denominator=den_Gd  SampleTime=Ts
  Discrete Derivative : simulink/Discrete/Discrete Derivative  gainval=1.0  ICPrevScaledInput=0.0  InputProcessing=Columns as channels (frame based)  OutMin=[]  OutMax=[]  OutDataType=fixdt(1, 16)  OutScaling=2^-10  DoSatur=off
  Display : Display
  Display1 : Display
  Encoder : arduinosensorlib/Encoder  InputA=2  InputB=20  Mode=No reset  SampleTime=-1
  Gain1 : Gain  Gain=encoder_scale
  Gain2 : Gain  Gain=60/(2*pi)
  Out1 : Outport
  wires:
  Gain1/1 -> Gain2/1, Display/1, Data Type Conversion1/1
  Encoder/1 -> Discrete Derivative/1
  Gain2/1 -> Display1/1
  Discrete Derivative/1 -> Gain1/1
  Discrete Transfer Fcn/1 -> Out1/1  "W(rad/s)"
  Data Type Conversion1/1 -> Discrete Transfer Fcn/1

== stateflow chart project_Auto_final/Chart ==
  state AD_mode [commented out]
    en:
    flag1 = sw1, flag2 = sw2;
    du:
    mode = 1;
  state AD_mode1
    en:
    flag1 = sw1, flag2 = sw2;
    du:
    mode = 1;
  state mode_off [commented out]
    en:
    flag1 = sw1, flag2 = sw2;
    du:
    mode = 0;
  state mode_off1
    en:
    flag1 = sw1, flag2 = sw2;
    du:
    mode = 0;
  state DMS_mode [commented out]
    en:
    flag1 = sw1, flag2 = sw2;
    du:
    mode = 2;
  state DMS_mode1
    en:
    flag1 = sw1, flag2 = sw2;
    du:
    mode = 2;
  mode_off -> AD_mode [commented out] : [flag1 ~= sw1]
  mode_off1 -> AD_mode1 : [flag1 ~= sw1]
  AD_mode1 -> DMS_mode1 : [flag1 ~= sw1]
  AD_mode -> mode_off [commented out] : [flag1 ~= sw1 || flag2 ~= sw2]
  (default) -> mode_off [commented out]
  (default) -> mode_off1
  DMS_mode -> mode_off [commented out] : [flag2 ~=  sw2 || flag1 ~= sw1]
  mode_off -> DMS_mode [commented out] : [flag2 ~= sw2]
  DMS_mode1 -> mode_off1 : [[flag1 ~= sw1]]
  data: sw1 input; sw2 input; mode output; flag1 local; flag2 local
